simulink model "work3"  (R2026a)
settings: Solver=ode45  StopTime=8  RelTol=1e-8  AbsTol=1e-10
settings Model: Creator=m  LastModifiedBy=m

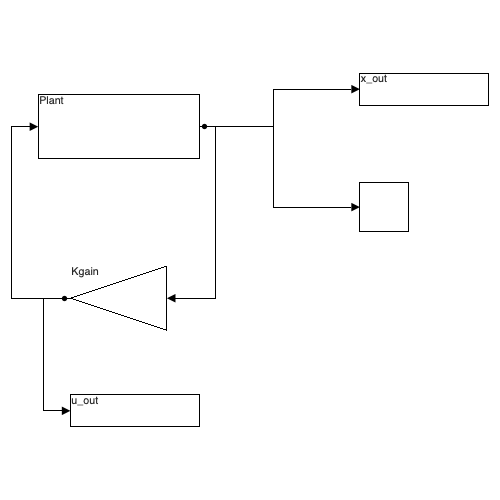
[thumbnail: Simulink's stored preview of the top-level diagram]
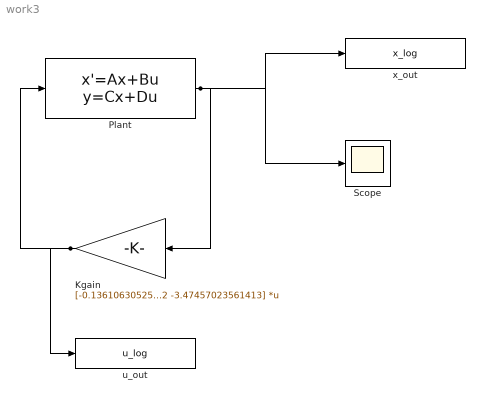
== system work3 ==
  Kgain : Gain  Gain=[-0.13610630525282 -3.47457023561413]  Multiplication=Matrix(K*u)
  Plant : StateSpace  A=[0 1;-2 5]  B=[0;3]  C=[1 0;0 1]  D=[0;0]  InitialCondition=[1;0]
  Scope : Scope
  u_out : ToWorkspace  VariableName=u_log  SaveFormat=Timeseries  SampleTime=-1
  x_out : ToWorkspace  VariableName=x_log  SaveFormat=Timeseries  SampleTime=-1
  wires:
  Plant/1 -> Kgain/1, x_out/1, Scope/1
  Kgain/1 -> Plant/1, u_out/1
